simulink model "perturbandobserve_battcharge"  (R2023a)
settings: Solver=VariableStepAuto  StartTime=0.0  StopTime=10.0  RelTol=1e-3
libraries: simulink x2, spsMeanLib x1
settings Model: Creator=gabrielcrisan  LastModifiedBy=gabrielcrisan

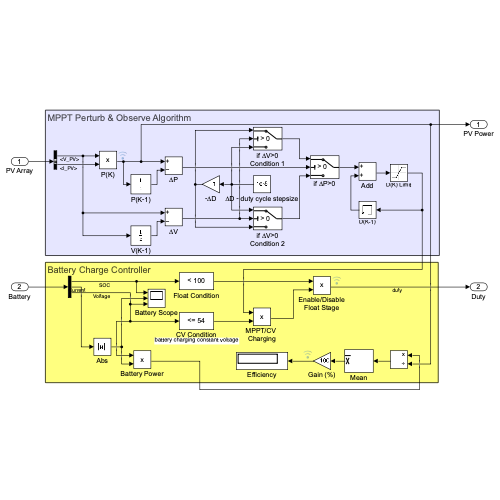
[thumbnail: Simulink's stored preview of the top-level diagram]
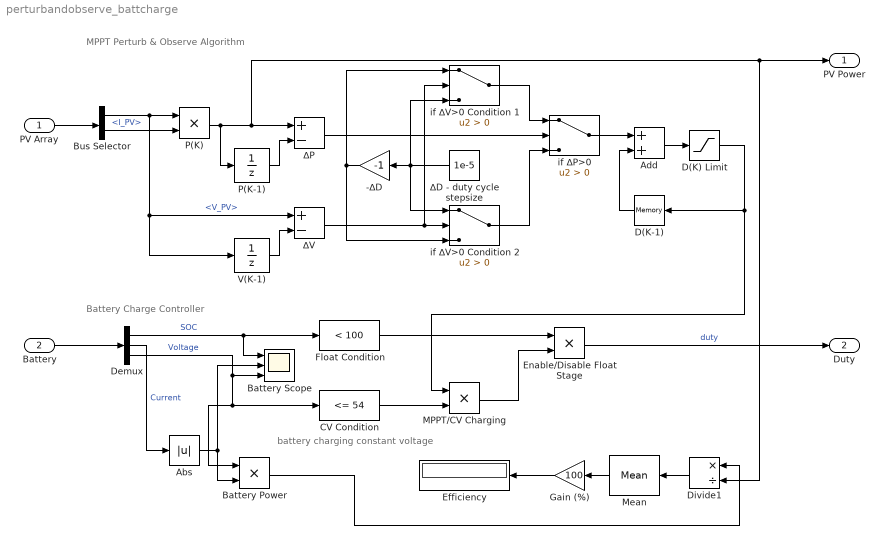
== system perturbandobserve_battcharge ==
  note: battery charging constant voltage
  note: MPPT Perturb & Observe Algorithm
  note: Battery Charge Controller
  PV Array : Inport
  Battery : Inport  Port=2
  -∆D : Gain  Gain=-1
  Abs : Abs  SaturateOnIntegerOverflow=off
  Add : Sum
  Battery Power : Product
  Battery Scope : Scope  NumInputPorts=3
  Bus Selector : BusSelector  OutputSignals=V_PV,I_PV
  CV Condition : simulink/Logic and Bit Operations/Compare To Constant  relop=<=  const=54  OutDataTypeStr=boolean
  D(K) Limit : Saturate  UpperLimit=0.6  LowerLimit=0.4
  D(K-1) : Memory  InitialCondition=0.5  InheritSampleTime=on  LinearizeMemory=on  LinearizeAsDelay=on
  Demux : Demux  Outputs=3
  Divide1 : Product  Inputs=*/
  Efficiency : Display
  Enable/Disable Float Stage : Product
  Float Condition : simulink/Logic and Bit Operations/Compare To Constant  relop=<  const=100  OutDataTypeStr=boolean
  Gain (%) : Gain  Gain=100
  MPPT/CV Charging : Product
  Mean : spsMeanLib/Mean  Freq=1  Vinit=0  Ts=0
  P(K) : Product
  P(K-1) : UnitDelay  SampleTime=-1  HasFrameUpgradeWarning=on
  V(K-1) : UnitDelay  SampleTime=-1  HasFrameUpgradeWarning=on
  if ∆P>0 : Switch  Criteria=u2 > Threshold  SaturateOnIntegerOverflow=off  InputSameDT=off
  if ∆V>0 Condition 1 : Switch  Criteria=u2 > Threshold  SaturateOnIntegerOverflow=off  InputSameDT=off
  if ∆V>0 Condition 2 : Switch  Criteria=u2 > Threshold  SaturateOnIntegerOverflow=off  InputSameDT=off
  ∆D - duty cycle stepsize : Constant  Value=1e-5
  ∆P : Sum  Inputs=+-
  ∆V : Sum  Inputs=+-
  PV Power : Outport  VectorParamsAs1DForOutWhenUnconnected=off
  Duty : Outport  Port=2  VectorParamsAs1DForOutWhenUnconnected=off
  wires:
  Mean/1 -> Gain (%)/1
  PV Array/1 -> Bus Selector/1
  Add/1 -> D(K) Limit/1
  if ∆V>0 Condition 1/1 -> if ∆P>0/1
  if ∆P>0/1 -> Add/1
  ∆P/1 -> if ∆P>0/2
  if ∆V>0 Condition 2/1 -> if ∆P>0/3
  Abs/1 -> Battery Scope/2, Battery Power/2
  Battery/1 -> Demux/1
  Bus Selector/1 -> ∆V/1, V(K-1)/1, P(K)/1  "<V_PV>"
  D(K) Limit/1 -> D(K-1)/1, MPPT/CV Charging/1
  Divide1/1 -> Mean/1
  CV Condition/1 -> MPPT/CV Charging/2
  V(K-1)/1 -> ∆V/2
  Bus Selector/2 -> P(K)/2  "<I_PV>"
  ∆V/1 -> if ∆V>0 Condition 2/2, if ∆V>0 Condition 1/2
  Enable/Disable Float Stage/1 -> Duty/1  "duty"
  P(K)/1 -> ∆P/1, Divide1/2, PV Power/1, P(K-1)/1
  Gain (%)/1 -> Efficiency/1
  Battery Power/1 -> Divide1/1
  P(K-1)/1 -> ∆P/2
  ∆D - duty cycle stepsize/1 -> if ∆V>0 Condition 2/1, -∆D/1, if ∆V>0 Condition 1/3
  Demux/1 -> Float Condition/1, Battery Scope/1  "SOC"
  D(K-1)/1 -> Add/2
  Float Condition/1 -> Enable/Disable Float Stage/1
  MPPT/CV Charging/1 -> Enable/Disable Float Stage/2
  -∆D/1 -> if ∆V>0 Condition 2/3, if ∆V>0 Condition 1/1
  Demux/2 -> Abs/1  "Current"
  Demux/3 -> Battery Scope/3, CV Condition/1, Battery Power/1  "Voltage"
